simulink model "pacemaker"  (R2022b)
settings: Solver=FixedStepAuto  StartTime=0.0  StopTime=10.0  FixedStep=1e-3  RelTol=1e-3  EnableMultiTasking=on
undefined symbols (not defined in the file): a, A0, A1, b, c, D0, D1, D10, D11, D12, D13, D2, D3, D4, D5, D6, D7, D8, D9, PTA0, PTA1, PTA2, PTB2, PTB23, PTB3, PTB9, PTC16, PTC17, PTC2, PTC3, PTC4, PTD0, PTD1, PTD2, PTD3
libraries: frdmk64flib x21, simulink x2, etargetslib x2, dspstat3 x1, hdlsllib x1
settings Model: ExtModeTrigDuration=5  Creator=arnur  LastModifiedBy=arnur
settings SolverCC: AlgebraicLoopSolver=TrustRegion
settings OptimizationCC: EnhancedBackFolding=on  PassReuseOutputArgsAs=Individual arguments  ZeroExternalMemoryAtStartup=off  ZeroInternalMemoryAtStartup=off  MaxStackSize=64  OptimizeBlockOrder=speed  DifferentSizesBufferReuse=on  OptimizationCustomize=off  EfficientTunableParamExpr=on
settings DebuggingCC: ParameterTunabilityLossMsg=error  UnconnectedInputMsg=warning  UnconnectedOutputMsg=warning  UnconnectedLineMsg=warning
settings HardwareCC: ProdBitPerPointer=32  ProdBitPerSizeT=32  ProdBitPerPtrDiffT=32  ProdLargestAtomicInteger=Long  ProdLargestAtomicFloat=Double  ProdWordSize=32  ProdHWDeviceType=ARM Compatible->ARM Cortex
settings ModelReferenceCC: EnableRefExpFcnMdlSchedulingChecks=on
settings SFSimCC: MATLABDynamicMemAlloc=off
settings RTWCC: Description=Embedded Coder  SystemTargetFile=ert.tlc  HardwareBoard=NXP FRDM-K64F  TLCOptions="-aInlineSetEventsForThisBaseRateFcn=TLC_FALSE -aSuppressMultiTaskScheduler=TLC_FALSE  -aRateBasedStepFcn=0"  TemplateMakefile=ert_default_tmf  Toolchain=GNU Tools for ARM Embedded Processors
settings CodeAppCC: ForceParamTrailComments=on  IgnoreCustomStorageClasses=off  OperatorAnnotations=on  SimulinkDataObjDesc=on  SFDataObjDesc=on  InsertBlockDesc=on

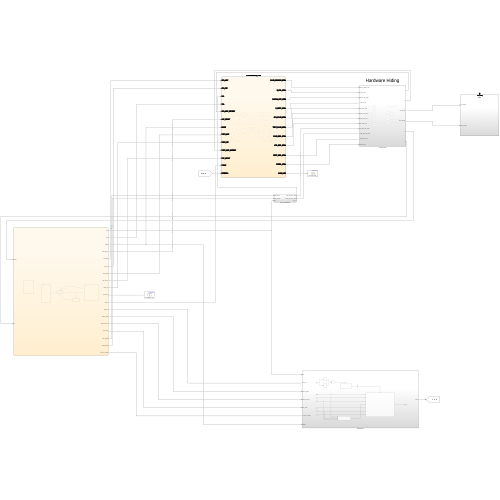
[thumbnail: Simulink's stored preview of the top-level diagram]
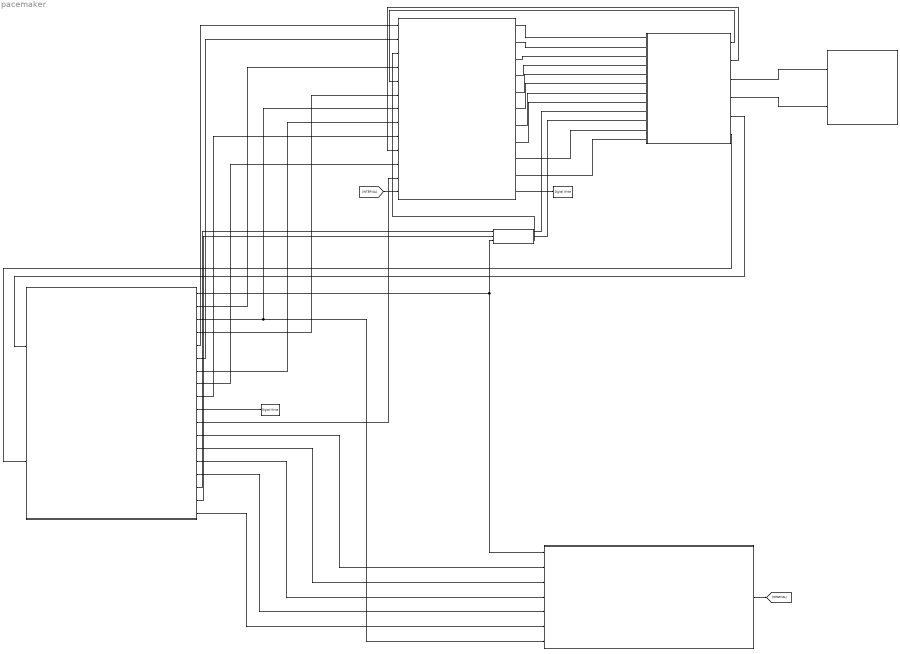
== system pacemaker ==
  note: Hardware Hiding
  Chart : Stateflow chart  TreatAsAtomicUnit=on
      settings: PortSchema="{\"entries\":[{\"content\":{\"sides\":[{\"content\":{\"connectorIds\":[\"In2\",\"In1\"]},\"type\":\"ConnectorPlacement.EquallySpacedRectSide\",\"uuid\":\"bc218187-1f13-41e7-927e-dd226419d8de\"},{\"content\":{\"connectorIds\":[\"Out1\",\"Out2\",\"Out3\",\"Out4\",\"Out5\",\"Out6\",\"Out7\",\"Out8\",\"Out9\",\"Out10\",\"Out11\",\"Out12\",\"Out13\",\"Out14\",\"Out15\",\"Out16\",\"Out17\",\"Out18\"],\"side\":\"RIGHT\"},\"type\":\"ConnectorPlacement.EquallySpacedRectSide\",\"uuid\":\"24412552-eff0-4bdb-8788-4cded0bceaa8\"},{\"content\":{\"connectorIds\":[],\"side\":\"TOP\"},\"type\":\"ConnectorPlacement.EquallySpacedRectSide\",\"uuid\":\"ae10373c-f6da-40d4-8510-ccb7acfbe125\"}]},\"type\":\"ConnectorPlacement.EquallySpacedConnector\",\"uuid\":\"32cdb14c-4a7f-42e8-a7b0-e0b40f5ef528\"}],\"packageUris\":[\"http://schema.mathworks.com/mf0/Connector/R2020b\"],\"version\":\"1.0\"}"
  Digital Write : frdmk64flib/Digital Write  Whichpin=GREEN_LED
  Digital Write1 : frdmk64flib/Digital Write  Whichpin=BLUE_LED
  Hardware Hiding : Subsystem
  INPUT_CONVERSION : Subsystem
  PACEMAKER_FSM : Stateflow chart  TreatAsAtomicUnit=on
  Rate Adaptivity : Subsystem
  Subsystem : Subsystem
  wires:
  Hardware Hiding/1(Output4) -> PACEMAKER_FSM/5(ATR_CMP_DETECT)
  Hardware Hiding/2(Output10) -> PACEMAKER_FSM/10(VENT_CMP_DETECT)
  Chart/5(ATR_AMP) -> PACEMAKER_FSM/1(ATR_AMP)
  Chart/9(VENT_PW) -> PACEMAKER_FSM/9(VENT_PW)
  Chart/8(VRP_DELAY) -> PACEMAKER_FSM/11(VRP_DELAY)
  PACEMAKER_FSM/2(Z_ATR_CTRL) -> Hardware Hiding/2(Z_ATR_CTRL)
  Chart/6(ATR_PW) -> PACEMAKER_FSM/2(ATR_PW)
  PACEMAKER_FSM/8(ATR_GND_CTRL) -> Hardware Hiding/8(ATR_GND_CTRL)
  Chart/7(VENT_AMP) -> PACEMAKER_FSM/8(VENT_AMP)
  Chart/1(LRL) -> INPUT_CONVERSION/3(LRL), Rate Adaptivity/1(LRL)
  Chart/2(URL) -> PACEMAKER_FSM/4(URL)
  PACEMAKER_FSM/5(ATR_PACE_CTRL) -> Hardware Hiding/5(ATR_PACE_CTRL)
  Chart/4(ARP_DELAY) -> PACEMAKER_FSM/6(ARP_DELAY)
  PACEMAKER_FSM/3(PACING_REF_PWM) -> Hardware Hiding/3(PACING_REF_PWM)
  PACEMAKER_FSM/6(VENT_PACE_CTRL) -> Hardware Hiding/6(VENT_PACE_CTRL)
  PACEMAKER_FSM/1(PACE_CHARGE_CTRL) -> Hardware Hiding/1(PACE_CHARGE_CTRL)
  Chart/3(MODE) -> PACEMAKER_FSM/7(MODE), Rate Adaptivity/7(MODE)
  PACEMAKER_FSM/9(VENT_GND_CTRL) -> Hardware Hiding/11(VENT_GND_CTRL)
  PACEMAKER_FSM/4(Z_VENT_CTRL) -> Hardware Hiding/4(Z_VENT_CTRL)
  PACEMAKER_FSM/7(PACE_GND_CTRL) -> Hardware Hiding/7(PACE_GND_CTRL)
  PACEMAKER_FSM/10(FRTND_CTRL) -> Hardware Hiding/12(FRTND_CTRL)
  Chart/10(green_LED) -> Digital Write/1
  Chart/11(PVARP) -> PACEMAKER_FSM/12(PVARP)
  Chart/12(MAX_SR) -> Rate Adaptivity/2(MAX_SR)
  Chart/13(REACT_TIME) -> Rate Adaptivity/3(REACT_TIME)
  Chart/14(RESP_FACTOR) -> Rate Adaptivity/4(RESP_FACTOR)
  Chart/15(REC_TIME) -> Rate Adaptivity/5(REC_TIME)
  Chart/16(ATR_SENSE) -> INPUT_CONVERSION/1(ATR_SENSE)
  Chart/17(VENT_SENSE) -> INPUT_CONVERSION/2(VENT_SENSE)
  Chart/18(ACTIVITY_THRES) -> Rate Adaptivity/6(ACTIVITY_THRES)
  Hardware Hiding/3(ATR_SIGNAL) -> Subsystem/1(ATR_SIGNAL)
  Hardware Hiding/4(VENT_SIGNAL) -> Subsystem/2(VENT_SIGNAL)
  INPUT_CONVERSION/1(ATR_CMP_REF_PWM) -> Hardware Hiding/9(ATR_CMP_REF_PWM)
  INPUT_CONVERSION/2(VENT_CMP_REF_PWM) -> Hardware Hiding/10(VENT_CMP_REF_PWM)
  Rate Adaptivity/1(interval) -> [INTERVAL]
  [INTERVAL] -> PACEMAKER_FSM/13(INTERVAL)
  PACEMAKER_FSM/11(BLUE_LED) -> Digital Write1/1
  INPUT_CONVERSION/3(LRL_P) -> PACEMAKER_FSM/3(LRL)
  Hardware Hiding/5(Output1) -> Chart/2(Status)
  Hardware Hiding/6(Output2) -> Chart/1(Rx)

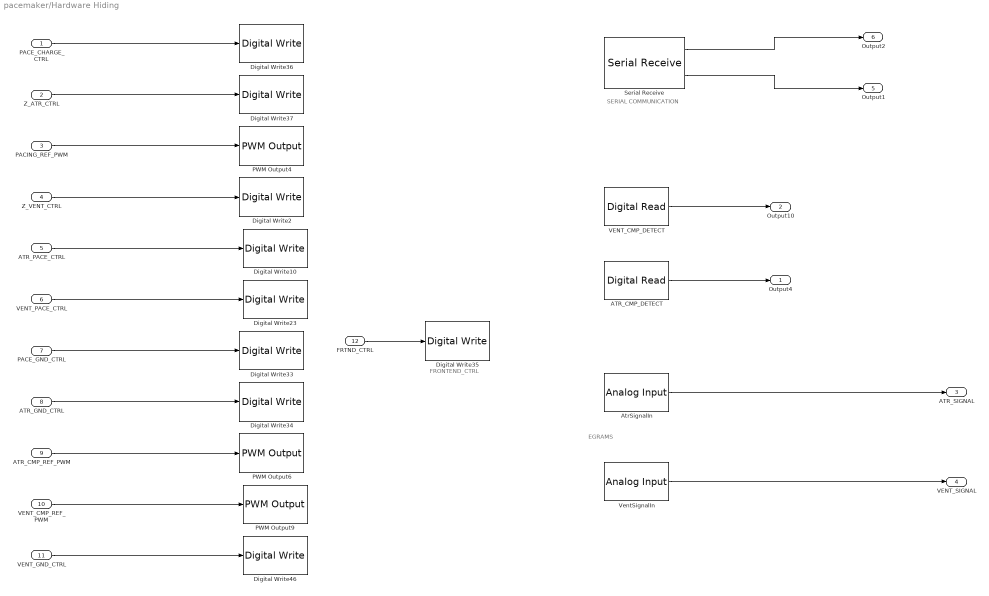
== system pacemaker/Hardware Hiding ==
  note: EGRAMS
  note: SERIAL COMMUNICATION
  note: FRONTEND_CTRL
  PACE_CHARGE_CTRL : Inport
  Z_ATR_CTRL : Inport  Port=2
  PACING_REF_PWM : Inport  Port=3
  Z_VENT_CTRL : Inport  Port=4
  ATR_PACE_CTRL : Inport  Port=5
  VENT_PACE_CTRL : Inport  Port=6
  PACE_GND_CTRL : Inport  Port=7
  ATR_GND_CTRL : Inport  Port=8
  ATR_CMP_REF_PWM : Inport  Port=9
  VENT_CMP_REF_PWM : Inport  Port=10
  VENT_GND_CTRL : Inport  Port=11
  FRTND_CTRL : Inport  Port=12  OutDataTypeStr=boolean  LockScale=on
  ATR_CMP_DETECT : frdmk64flib/Digital Read  Whichpin=PTC16 (D0)  SampleTime=-1
  AtrSignalIn : frdmk64flib/Analog Input  Whichpin=PTB2 (A0)  SampleTime=-1
  Digital Write10 : frdmk64flib/Digital Write  Whichpin=PTA0 (D8)
  Digital Write2 : frdmk64flib/Digital Write  Whichpin=PTC3 (D7)
  Digital Write23 : frdmk64flib/Digital Write  Whichpin=PTC4 (D9)
  Digital Write33 : frdmk64flib/Digital Write  Whichpin=PTD0 (D10)
  Digital Write34 : frdmk64flib/Digital Write  Whichpin=PTD2 (D11)
  Digital Write35 : frdmk64flib/Digital Write  Whichpin=PTD1 (D13)
  Digital Write36 : frdmk64flib/Digital Write  Whichpin=PTB9 (D2)
  Digital Write37 : frdmk64flib/Digital Write  Whichpin=PTB23 (D4)
  Digital Write46 : frdmk64flib/Digital Write  Whichpin=PTD3 (D12)
  PWM Output4 : frdmk64flib/PWM Output  Whichpin=PTA2 (D5)  InitialFrequency=2000  InitialDutyCycle=0
  PWM Output6 : frdmk64flib/PWM Output  Whichpin=PTC2 (D6)  InitialFrequency=2000  InitialDutyCycle=0
  PWM Output9 : frdmk64flib/PWM Output  Whichpin=PTA1 (D3)  InitialFrequency=2000  InitialDutyCycle=0
  Serial Receive : frdmk64flib/Serial Receive  SCIModule=0  Baudrate=uint32(9600)  Parity=None  StopBits=1  HardwareFlowControl=None  ByteOrder=LittleEndian  DataType=uint8  DataLength=49  BlockingMode=off  OutputStatus=on  SampleTime=-1
  VENT_CMP_DETECT : frdmk64flib/Digital Read  Whichpin=PTC17 (D1)  SampleTime=-1
  VentSignalIn : frdmk64flib/Analog Input  Whichpin=PTB3 (A1)  SampleTime=-1
  Output4 : Outport
  Output10 : Outport  Port=2
  ATR_SIGNAL : Outport  Port=3
  VENT_SIGNAL : Outport  Port=4
  Output1 : Outport  Port=5
  Output2 : Outport  Port=6
  wires:
  VENT_GND_CTRL/1 -> Digital Write46/1
  Z_VENT_CTRL/1 -> Digital Write2/1
  VENT_PACE_CTRL/1 -> Digital Write23/1
  ATR_CMP_REF_PWM/1 -> PWM Output6/1
  VENT_CMP_REF_PWM/1 -> PWM Output9/1
  PACE_CHARGE_CTRL/1 -> Digital Write36/1
  Z_ATR_CTRL/1 -> Digital Write37/1
  ATR_PACE_CTRL/1 -> Digital Write10/1
  PACE_GND_CTRL/1 -> Digital Write33/1
  ATR_GND_CTRL/1 -> Digital Write34/1
  PACING_REF_PWM/1 -> PWM Output4/1
  ATR_CMP_DETECT/1 -> Output4/1
  VENT_CMP_DETECT/1 -> Output10/1
  FRTND_CTRL/1 -> Digital Write35/1
  VentSignalIn/1 -> VENT_SIGNAL/1
  AtrSignalIn/1 -> ATR_SIGNAL/1
  Serial Receive/1 -> Output2/1
  Serial Receive/2 -> Output1/1

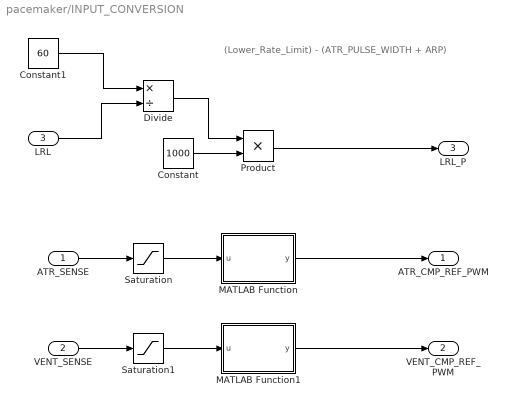
== system pacemaker/INPUT_CONVERSION ==
  note: (Lower_Rate_Limit) - (ATR_PULSE_WIDTH + ARP)
  ATR_SENSE : Inport
  VENT_SENSE : Inport  Port=2
  LRL : Inport  Port=3  OutDataTypeStr=uint16
  Constant : Constant  Value=1000  OutDataTypeStr=double
  Constant1 : Constant  Value=60  OutDataTypeStr=double
  Divide : Product  Inputs=*/  OutDataTypeStr=double
  MATLAB Function : MATLAB Function  TreatAsAtomicUnit=on
  MATLAB Function1 : MATLAB Function  TreatAsAtomicUnit=on
  Product : Product  OutDataTypeStr=double
  Saturation : Saturate  UpperLimit=4  LowerLimit=0.65  OutDataTypeStr=double
  Saturation1 : Saturate  UpperLimit=4  LowerLimit=0.65  OutDataTypeStr=double
  ATR_CMP_REF_PWM : Outport
  VENT_CMP_REF_PWM : Outport  Port=2
  LRL_P : Outport  Port=3  OutDataTypeStr=double
  wires:
  ATR_SENSE/1 -> Saturation/1
  Saturation/1 -> MATLAB Function/1(u)
  MATLAB Function/1(y) -> ATR_CMP_REF_PWM/1
  MATLAB Function1/1(y) -> VENT_CMP_REF_PWM/1
  VENT_SENSE/1 -> Saturation1/1
  Saturation1/1 -> MATLAB Function1/1(u)
  Product/1 -> LRL_P/1
  Constant/1 -> Product/2
  LRL/1 -> Divide/2
  Divide/1 -> Product/1
  Constant1/1 -> Divide/1

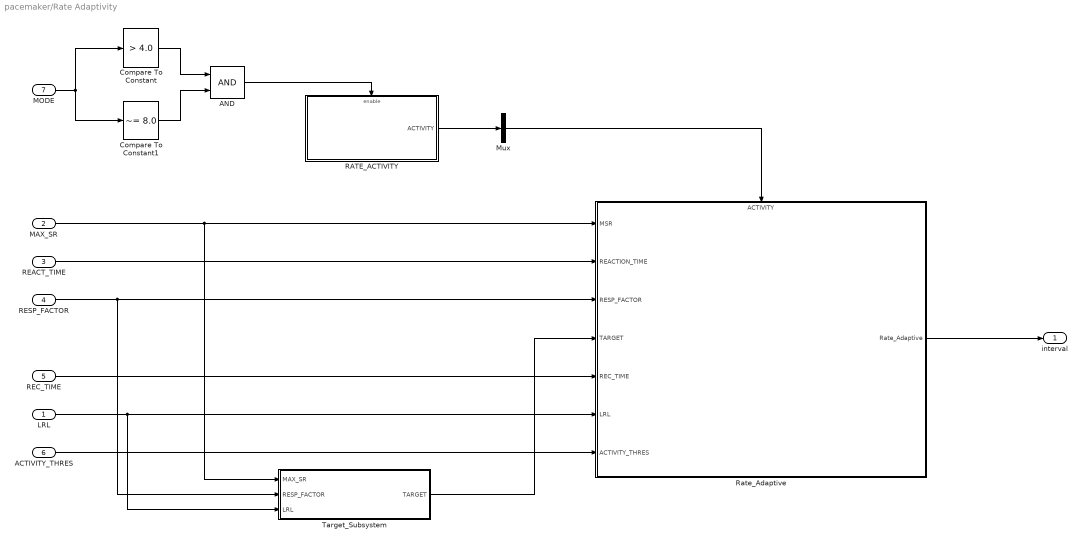
== system pacemaker/Rate Adaptivity ==
  LRL : Inport
  MAX_SR : Inport  Port=2
  REACT_TIME : Inport  Port=3
  RESP_FACTOR : Inport  Port=4
  REC_TIME : Inport  Port=5
  ACTIVITY_THRES : Inport  Port=6  OutDataTypeStr=double
  MODE : Inport  Port=7
  AND : Logic  IconShape=distinctive  AllPortsSameDT=off  OutDataTypeStr=boolean
  Compare To Constant : simulink/Logic and Bit Operations/Compare To Constant  relop=>  const=4.0  OutDataTypeStr=boolean
  Compare To Constant1 : simulink/Logic and Bit Operations/Compare To Constant  relop=~=  const=8.0  OutDataTypeStr=boolean
  Mux : Mux  Inputs=1
  RATE_ACTIVITY : Subsystem
  Rate_Adaptive : Subsystem
      settings: PortSchema="{\"entries\":[{\"content\":{\"sides\":[{\"content\":{\"connectorIds\":[\"In1\",\"In2\",\"In3\",\"In4\",\"In5\",\"In6\",\"In7\"]},\"type\":\"ConnectorPlacement.EquallySpacedRectSide\",\"uuid\":\"ecef5992-6168-4615-8079-152f4001d897\"},{\"content\":{\"connectorIds\":[\"Out1\"],\"side\":\"RIGHT\"},\"type\":\"ConnectorPlacement.EquallySpacedRectSide\",\"uuid\":\"4b0443a4-3c4f-432b-8acf-b8853e3911f3\"},{\"content\":{\"connectorIds\":[\"In8\"],\"side\":\"TOP\"},\"type\":\"ConnectorPlacement.EquallySpacedRectSide\",\"uuid\":\"9eb25122-da38-4088-8f00-2d2dff5efbee\"},{\"content\":{\"connectorIds\":[],\"side\":\"BOTTOM\"},\"type\":\"ConnectorPlacement.EquallySpacedRectSide\",\"uuid\":\"f562ad64-64af-4bdb-b61f-82ac1a60a400\"}]},\"type\":\"ConnectorPlacement.EquallySpacedConnector\",\"uuid\":\"02b21474-b9be-4120-8392-47ed1544c592\"}],\"packageUris\":[\"http://schema.mathworks.com/mf0/Connector/R2020b\"],\"version\":\"1.0\"}"
  Target_Subsystem : Subsystem
  interval : Outport
  wires:
  REC_TIME/1 -> Rate_Adaptive/5(REC_TIME)
  Target_Subsystem/1(TARGET) -> Rate_Adaptive/4(TARGET)
  REACT_TIME/1 -> Rate_Adaptive/2(REACTION_TIME)
  Rate_Adaptive/1(Rate_Adaptive) -> interval/1
  RESP_FACTOR/1 -> Rate_Adaptive/3(RESP_FACTOR), Target_Subsystem/2(RESP_FACTOR)
  LRL/1 -> Target_Subsystem/3(LRL), Rate_Adaptive/6(LRL)
  MAX_SR/1 -> Target_Subsystem/1(MAX_SR), Rate_Adaptive/1(MSR)
  ACTIVITY_THRES/1 -> Rate_Adaptive/7(ACTIVITY_THRES)
  AND/1 -> RATE_ACTIVITY/Enable
  Mux/1 -> Rate_Adaptive/8(ACTIVITY)
  Compare To Constant/1 -> AND/1
  Compare To Constant1/1 -> AND/2
  RATE_ACTIVITY/1(ACTIVITY) -> Mux/1
  MODE/1 -> Compare To Constant1/1, Compare To Constant/1

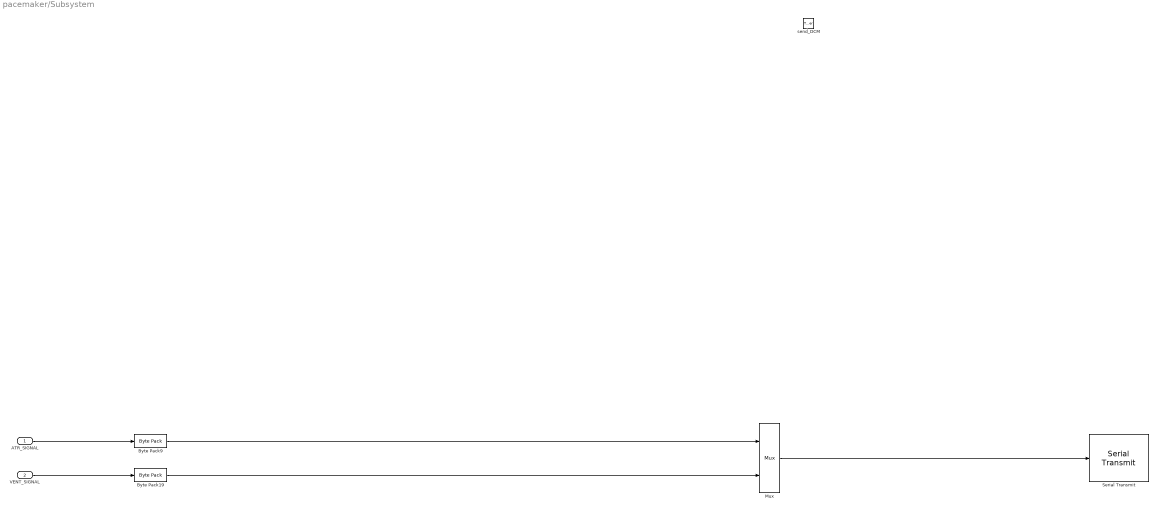
== system pacemaker/Subsystem ==
  ATR_SIGNAL : Inport
  VENT_SIGNAL : Inport  Port=2
  send_DCM : TriggerPort  TriggerType=function-call  IsSimulinkFunction=on  FunctionName=send_DCM  VariantControl=Variant
  Byte Pack19 : etargetslib/Byte Pack  datatypes={'double'}  byteAlign=1
  Byte Pack9 : etargetslib/Byte Pack  datatypes={'double'}  byteAlign=1
  Mux : Mux  Inputs=2
  Serial Transmit : frdmk64flib/Serial Transmit  SCIModule=0  Baudrate=uint32(9600)  Parity=None  StopBits=1  HardwareFlowControl=None  ByteOrder=LittleEndian  BlockingMode=on  OutputStatus=off
  wires:
  Mux/1 -> Serial Transmit/1
  ATR_SIGNAL/1 -> Byte Pack9/1
  VENT_SIGNAL/1 -> Byte Pack19/1
  Byte Pack9/1 -> Mux/1
  Byte Pack19/1 -> Mux/2

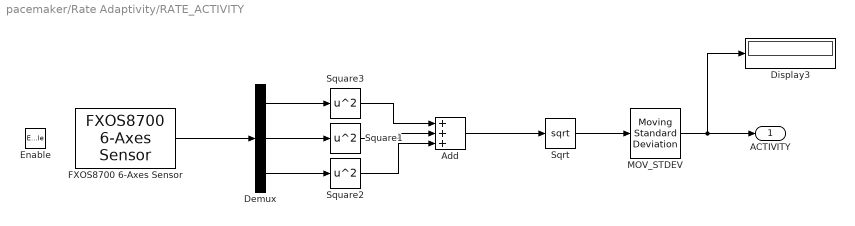
== system pacemaker/Rate Adaptivity/RATE_ACTIVITY ==
  Enable : EnablePort
  Add : Sum  Inputs=+++
  Demux : Demux  Outputs=3
  Display3 : Display
  FXOS8700 6-Axes Sensor : frdmk64flib/FXOS8700 6-Axes Sensor  Activesensor=Accelerometer only  ODR=800Hz  HybridODR=400Hz  Accelfullrange=-4g to +4g  SampleTime=-1
  MOV_STDEV : dspstat3/Moving Standard Deviation  Method=Sliding window  ForgettingFactorPort=off  SpecifyWindowLength=on  WindowLength=156  OverlapLength=155  AllowArbitraryInputLength=off  ForgettingFactor=0.9  SimulateUsing=Code generation
  Sqrt : Sqrt
  Square1 : Math  Operator=square  OutDataTypeStr=double
  Square2 : Math  Operator=square  OutDataTypeStr=double
  Square3 : Math  Operator=square  OutDataTypeStr=double
  ACTIVITY : Outport
  wires:
  FXOS8700 6-Axes Sensor/1 -> Demux/1
  Demux/3 -> Square2/1
  Square1/1 -> Add/2
  Add/1 -> Sqrt/1
  Demux/2 -> Square1/1
  Square3/1 -> Add/1
  Square2/1 -> Add/3
  Demux/1 -> Square3/1
  Sqrt/1 -> MOV_STDEV/1
  MOV_STDEV/1 -> Display3/1, ACTIVITY/1

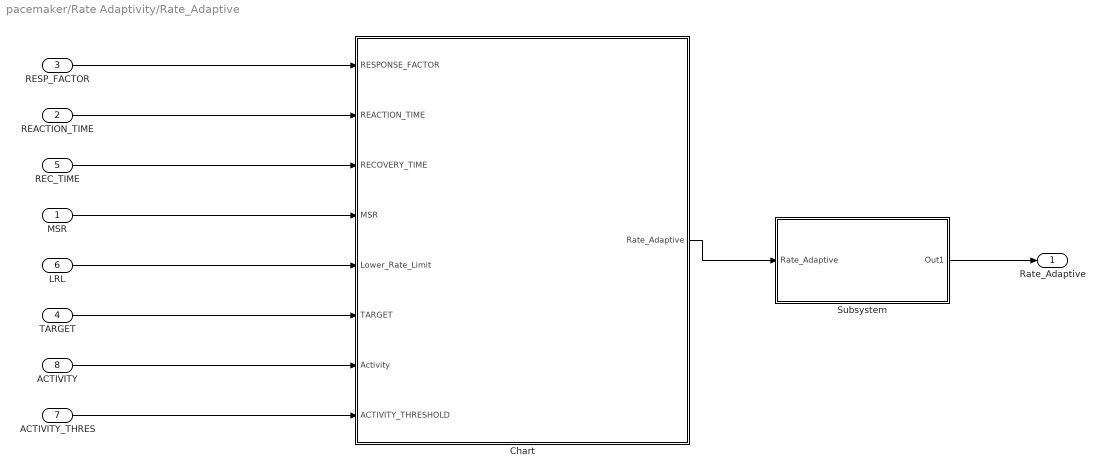
== system pacemaker/Rate Adaptivity/Rate_Adaptive ==
  MSR : Inport
  REACTION_TIME : Inport  Port=2
  RESP_FACTOR : Inport  Port=3
  TARGET : Inport  Port=4
  REC_TIME : Inport  Port=5
  LRL : Inport  Port=6
  ACTIVITY_THRES : Inport  Port=7
  ACTIVITY : Inport  Port=8
  Chart : Stateflow chart  TreatAsAtomicUnit=on
  Subsystem : Subsystem
  Rate_Adaptive : Outport
  wires:
  RESP_FACTOR/1 -> Chart/1(RESPONSE_FACTOR)
  REACTION_TIME/1 -> Chart/2(REACTION_TIME)
  REC_TIME/1 -> Chart/3(RECOVERY_TIME)
  ACTIVITY_THRES/1 -> Chart/8(ACTIVITY_THRESHOLD)
  MSR/1 -> Chart/4(MSR)
  LRL/1 -> Chart/5(Lower_Rate_Limit)
  TARGET/1 -> Chart/6(TARGET)
  ACTIVITY/1 -> Chart/7(Activity)
  Chart/1(Rate_Adaptive) -> Subsystem/1(Rate_Adaptive)
  Subsystem/1(Out1) -> Rate_Adaptive/1

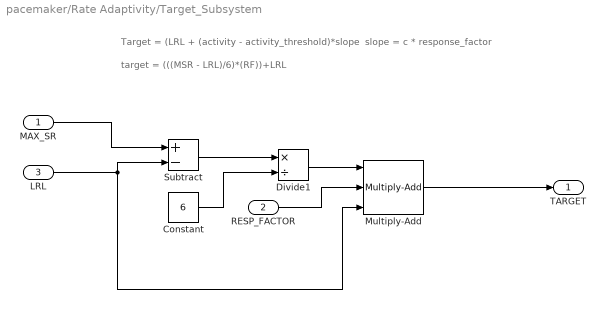
== system pacemaker/Rate Adaptivity/Target_Subsystem ==
  note: target = (((MSR - LRL)/6)*(RF))+LRL
  note: slope = c * response_factor
  note: Target = (LRL + (activity - activity_threshold)*slope
  MAX_SR : Inport
  RESP_FACTOR : Inport  Port=2
  LRL : Inport  Port=3
  Constant : Constant  Value=6
  Divide1 : Product  Inputs=*/
  Multiply-Add : hdlsllib/HDL Operations/Multiply-Add  Function=c+(a.*b)  datatype=uint16  RndMeth=Round  DoSatur=off  FMA=off
  Subtract : Sum  Inputs=+-
  TARGET : Outport  OutDataTypeStr=uint16
  wires:
  RESP_FACTOR/1 -> Multiply-Add/2
  Constant/1 -> Divide1/2
  MAX_SR/1 -> Subtract/1
  LRL/1 -> Subtract/2, Multiply-Add/3
  Divide1/1 -> Multiply-Add/1
  Multiply-Add/1 -> TARGET/1
  Subtract/1 -> Divide1/1

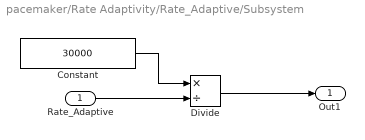
== system pacemaker/Rate Adaptivity/Rate_Adaptive/Subsystem ==
  Rate_Adaptive : Inport
  Constant : Constant  Value=30000  OutDataTypeStr=uint16
  Divide : Product  Inputs=*/
  Out1 : Outport  OutDataTypeStr=uint16
  wires:
  Constant/1 -> Divide/1
  Rate_Adaptive/1 -> Divide/2
  Divide/1 -> Out1/1

== matlab function pacemaker/INPUT_CONVERSION/MATLAB Function1 ==
  data: u input; y output
function y = fcn(u)

y = u./5.*100;

== matlab function pacemaker/INPUT_CONVERSION/MATLAB Function ==
  data: u input; y output
function y = fcn(u)

y = u./5.*100;

== stateflow chart pacemaker/Chart ==
  note: MODE
      | AOO: 1
      | AAI: 2
      | VVO: 3
      | VVI: 4
      | %RATE ADAPTIVE
      | AOOR: 5
      | AAIR: 6
      | VOOR: 7
      | VVIR: 8
  state INITIAL
    %initializing parameters
    entry:
    MODE = 5;
    LRL = 60;
    URL = 120;
    ARP_DELAY  =200;
    ATR_AMP = 3.5;
    VENT_AMP= 3.5;
    VRP_DELAY= 200;
    ATR_PW= 10;
    VENT_PW = 10;
    %
    PVARP = 200% uint_16
    MAX_SR = 120 % uint_16
    REACT_TIME = 30 %uint_8
    RESP_FACTOR = 16 %uint_8
    REC_TIME = 2 %uint_8
    ATR_SENSE = 3 %single
    VENT_SENSE = 3%single
    ACTIVITY_THRES = 0.2 % uint_8
    %
    green_LED = false;
  state SET_PARAM
    entry:
    MODE = typecast(Rx(3),'uint8');
    LRL = typecast(Rx(4:5),'uint16');
    URL =typecast(Rx(6:7),'uint16');
    ARP_DELAY  = typecast(Rx(8:9),'uint16');
    ATR_AMP = typecast(Rx(10:13),'single');
    VENT_AMP= typecast(Rx(14:17),'single');
    VRP_DELAY= typecast(Rx(18:19),'uint16');
    ATR_PW= typecast(Rx(20:21),'uint16');
    VENT_PW = typecast(Rx(22:23),'uint16');
    ATR_SENSE = typecast(Rx(24:27), 'single');
    VENT_SENSE = typecast(Rx(28:31), 'single');
    PVARP = typecast(Rx(32:33), 'uint16');
    MAX_SR = typecast(Rx(34:35), 'uint16');
    REACT_TIME = typecast(Rx(36:37),'uint16');
    RESP_FACTOR =  typecast(Rx(38:39),'uint16');
    REC_TIME =  typecast(Rx(40:41),'uint16');
    ACTIVITY_THRES =  typecast(Rx(42:49),'double');
    green_LED = false;
  state STANDBY
    % Wait for the inputs
  state ECHO_PARAM
    entry:
    send_DCM();
    green_LED = false;
  (default) -> INITIAL
  SET_PARAM -> STANDBY
  (junction 33) -> STANDBY [order 2]
  INITIAL -> STANDBY
  STANDBY -> (junction 33) : [Status==0]
  (junction 33) -> (junction 36) [order 1] : [Rx(1)==hex2dec('16')]
  (junction 36) -> SET_PARAM [order 2] : [Rx(2) == hex2dec('12')]
  (junction 36) -> ECHO_PARAM [order 1] : [Rx(2) == hex2dec('22')]
  ECHO_PARAM -> STANDBY
  data: Rx input uint8; Status input uint8 size=1; LRL output uint16; URL output uint16; MODE output uint8; ARP_DELAY output uint16; ATR_AMP output single; ATR_PW output uint16; VENT_AMP output single; VRP_DELAY output uint16; VENT_PW output uint16; green_LED output boolean; PVARP output uint16; MAX_SR output uint16; REACT_TIME output uint16; RESP_FACTOR output uint16; REC_TIME output uint16; ATR_SENSE output single; VENT_SENSE output single; ACTIVITY_THRES output double

== stateflow chart pacemaker/Rate Adaptivity/Rate_Adaptive/Chart ==
  state State1
    entry:
    Rate_Adaptive = Lower_Rate_Limit;
    %when activity is less than activity threshold the rate adaptive is equal to LRL
  state State3
    entry:
    Rate_Adaptive = TARGET;
    %If activity is continued then the rate adaptive will eventually reach the target rate
  state State2
    entry:
    Rate_Adaptive = Rate_Adaptive + Step_Up;
    %Rate adaptive is calculated using step size when activity is high
  state State5
    entry:
    Rate_Adaptive = Rate_Adaptive - Step_Down;
    %continue to decrease rate adaptive until LRL is reached
  state State4
    entry:
    Rate_Adaptive = Rate_Adaptive - Step_Up;
    %once the activty starts decreasing we need to decrease rate adaptive
  (default) -> State1 : {Step_Up = ceil((TARGET - Lower_Rate_Limit)/REACTION_TIME);
      | Step_Down = ceil((TARGET - Lower_Rate_Limit)/RECOVERY_TIME)}
  State1 -> State1 [order 1] : [Activity < ACTIVITY_THRESHOLD]
  State2 -> State2 [order 2] : after(1000,msec)[Rate_Adaptive <= TARGET]
  State3 -> State3 [order 2] : [Activity > ACTIVITY_THRESHOLD]
  State1 -> State2 [order 2] : [Activity >= ACTIVITY_THRESHOLD]
  State2 -> State3 [order 3] : [Rate_Adaptive >= TARGET]
  State3 -> State5 [order 1] : [Activity < ACTIVITY_THRESHOLD]
  State5 -> State1 [order 1] : [Rate_Adaptive <= Lower_Rate_Limit]
  State5 -> State2 [order 3] : [Activity >= ACTIVITY_THRESHOLD]
  State2 -> State4 [order 1] : [Activity < ACTIVITY_THRESHOLD]
  State4 -> State2 [order 1] : [Activity >= ACTIVITY_THRESHOLD]
  State4 -> State5 [order 2] : [after(1000,msec)]
  State5 -> State5 [order 2] : after(1000,msec)[Rate_Adaptive >= Lower_Rate_Limit]
  data: RESPONSE_FACTOR input; REACTION_TIME input; RECOVERY_TIME input; MSR input; Lower_Rate_Limit input; TARGET input; Activity input; ACTIVITY_THRESHOLD input; Rate_Adaptive output; Step_Up local uint16; Step_Down local uint16

== stateflow chart pacemaker/PACEMAKER_FSM ==
  note: VOOR
  note: AOOR
  state Charging_C22_and_Discharging_Blocking_Cap4
    entry:
    FRTND_CTRL= true;
    ATR_PACE_CTRL = false;
    VENT_PACE_CTRL= false;
    PACING_REF_PWM = (ATR_AMP*100)/5;
    PACE_CHARGE_CTRL = true;
    PACE_GND_CTRL = true;
    Z_ATR_CTRL = false;
    Z_VENT_CTRL = false;
    ATR_GND_CTRL = true;
    FRTND_CTRL= true;
    BLUE_LED = false;
  state Charging_C22_and_Discharging_Blocking_Cap5
    entry:
    ATR_PACE_CTRL = false;
    VENT_PACE_CTRL= false;
    PACING_REF_PWM = (VENT_AMP*100)/5;
    PACE_CHARGE_CTRL = true;
    PACE_GND_CTRL = true;
    Z_ATR_CTRL = false;
    Z_VENT_CTRL = false;
    %ATR_GND_CTRL = true;
    VENT_GND_CTRL = true;
  state Discharging_C22_into_AV__charge_C26
    entry:
    PACE_CHARGE_CTRL = false;
    PACE_GND_CTRL = true;
    ATR_PACE_CTRL = false;
    %ATR_GND_CTRL = false;
    Z_ATR_CTRL = false;
    Z_VENT_CTRL = false;
    VENT_GND_CTRL = false;
    VENT_PACE_CTRL = true;
  state Discharging_C22_into_AV__charge_C25
    entry:
    FRTND_CTRL= false;
    PACE_CHARGE_CTRL = false;
    PACE_GND_CTRL = true;
    ATR_PACE_CTRL = true;
    ATR_GND_CTRL = false;
    Z_ATR_CTRL = false;
    Z_VENT_CTRL = false;
    VENT_PACE_CTRL = false;
    FRTND_CTRL= false;
    BLUE_LED = true;
  note: VOO
  note: AOO
  state Charging_C22_and_Discharging_Blocking_Cap3
    entry:
    ATR_PACE_CTRL = false;
    VENT_PACE_CTRL= false;
    PACING_REF_PWM = (VENT_AMP*100)/5;
    PACE_CHARGE_CTRL = true;
    PACE_GND_CTRL = true;
    Z_ATR_CTRL = false;
    Z_VENT_CTRL = false;
    %ATR_GND_CTRL = true;
    VENT_GND_CTRL = true;
  state Discharging_C22_into_AV__charge_C24
    entry:
    PACE_CHARGE_CTRL = false;
    PACE_GND_CTRL = true;
    ATR_PACE_CTRL = false;
    %ATR_GND_CTRL = false;
    Z_ATR_CTRL = false;
    Z_VENT_CTRL = false;
    VENT_GND_CTRL = false;
    VENT_PACE_CTRL = true;
  state Charging_C22_and_Discharging_Blocking_Cap
    entry:
    ATR_PACE_CTRL = false;
    VENT_PACE_CTRL= false;
    PACING_REF_PWM = (ATR_AMP*100)/5;
    PACE_CHARGE_CTRL = true;
    PACE_GND_CTRL = true;
    Z_ATR_CTRL = false;
    Z_VENT_CTRL = false;
    ATR_GND_CTRL = true;
    BLUE_LED = false;
  state Discharging_C22_into_AV__charge_C21
    entry:
    PACE_CHARGE_CTRL = false;
    PACE_GND_CTRL = true;
    ATR_PACE_CTRL = true;
    ATR_GND_CTRL = false;
    Z_ATR_CTRL = false;
    Z_VENT_CTRL = false;
    VENT_PACE_CTRL = false;
    BLUE_LED = true;
  state Initial
    entry:
    BLUE_LED = true;
    FRTND_CTRL= false;
  note: AAI
  note: VVI
  state Charging_C22_and_Discharging_Blocking_Cap2
    entry:
    ATR_PACE_CTRL = false;
    VENT_PACE_CTRL= false;
    PACING_REF_PWM = (VENT_AMP*100)/5;
    PACE_CHARGE_CTRL = true;
    PACE_GND_CTRL = true;
    Z_ATR_CTRL = false;
    Z_VENT_CTRL = false;
    %ATR_GND_CTRL = true;
    VENT_GND_CTRL = true;
    FRTND_CTRL= true;
  state Discharging_C22_into_AV__charge_C23
    entry:
    PACE_CHARGE_CTRL = false;
    PACE_GND_CTRL = true;
    ATR_PACE_CTRL = false;
    %ATR_GND_CTRL = false;
    Z_ATR_CTRL = false;
    Z_VENT_CTRL = false;
    VENT_GND_CTRL = false;
    VENT_PACE_CTRL = true;
  state Charging_C22_and_Discharging_Blocking_Cap1
    entry:
    ATR_PACE_CTRL = false;
    VENT_PACE_CTRL= false;
    PACING_REF_PWM = (ATR_AMP*100)/5;
    PACE_CHARGE_CTRL = true;
    PACE_GND_CTRL = true;
    Z_ATR_CTRL = false;
    Z_VENT_CTRL = false;
    ATR_GND_CTRL = true;
    FRTND_CTRL= true;
  state Discharging_C22_into_AV__charge_C22
    entry:
    PACE_CHARGE_CTRL = false;
    PACE_GND_CTRL = true;
    ATR_PACE_CTRL = true;
    ATR_GND_CTRL = false;
    Z_ATR_CTRL = false;
    Z_VENT_CTRL = false;
    VENT_PACE_CTRL = false;
  note: VVIR
  state Charging_C22_and_Discharging_Blocking_Cap6
    entry:
    ATR_PACE_CTRL = false;
    VENT_PACE_CTRL= false;
    PACING_REF_PWM = (ATR_AMP*100)/5;
    PACE_CHARGE_CTRL = true;
    PACE_GND_CTRL = true;
    Z_ATR_CTRL = false;
    Z_VENT_CTRL = false;
    ATR_GND_CTRL = true;
    FRTND_CTRL= true;
  state Charging_C22_and_Discharging_Blocking_Cap7
    entry:
    ATR_PACE_CTRL = false;
    VENT_PACE_CTRL= false;
    PACING_REF_PWM = (VENT_AMP*100)/5;
    PACE_CHARGE_CTRL = true;
    PACE_GND_CTRL = true;
    Z_ATR_CTRL = false;
    Z_VENT_CTRL = false;
    %ATR_GND_CTRL = true;
    VENT_GND_CTRL = true;
    FRTND_CTRL= true;
  state Discharging_C22_into_AV__charge_C28
    entry:
    PACE_CHARGE_CTRL = false;
    PACE_GND_CTRL = true;
    ATR_PACE_CTRL = false;
    %ATR_GND_CTRL = false;
    Z_ATR_CTRL = false;
    Z_VENT_CTRL = false;
    VENT_GND_CTRL = false;
    VENT_PACE_CTRL = true;
  state Discharging_C22_into_AV__charge_C27
    entry:
    PACE_CHARGE_CTRL = false;
    PACE_GND_CTRL = true;
    ATR_PACE_CTRL = true;
    ATR_GND_CTRL = false;
    Z_ATR_CTRL = false;
    Z_VENT_CTRL = false;
    VENT_PACE_CTRL = false;
  note: AAIR
  Charging_C22_and_Discharging_Blocking_Cap4 -> Discharging_C22_into_AV__charge_C25 : [after ((INTERVAL - ATR_PW ),msec)]
  Charging_C22_and_Discharging_Blocking_Cap5 -> Discharging_C22_into_AV__charge_C26 : [after ((INTERVAL - VENT_PW ),msec)]
  Discharging_C22_into_AV__charge_C26 -> Initial [order 2] : [MODE~=7]
  Discharging_C22_into_AV__charge_C26 -> Charging_C22_and_Discharging_Blocking_Cap5 [order 1] : [after(VENT_PW,msec)]
  Initial -> Charging_C22_and_Discharging_Blocking_Cap4 [order 5] : [MODE==5]
  Discharging_C22_into_AV__charge_C25 -> Charging_C22_and_Discharging_Blocking_Cap4 [order 2] : [after(ATR_PW,msec)]
  Initial -> Charging_C22_and_Discharging_Blocking_Cap5 [order 1] : [MODE==7]
  Discharging_C22_into_AV__charge_C25 -> Initial [order 1] : [MODE~=5]
  Discharging_C22_into_AV__charge_C21 -> Initial [order 2] : [MODE~=1]
  Initial -> Discharging_C22_into_AV__charge_C24 [order 8] : [MODE==3]
  Charging_C22_and_Discharging_Blocking_Cap3 -> Discharging_C22_into_AV__charge_C24 : [after ((LRL - VENT_PW ),msec)]
  Charging_C22_and_Discharging_Blocking_Cap -> Discharging_C22_into_AV__charge_C21 : [after ((LRL - ATR_PW ),msec)]
  Discharging_C22_into_AV__charge_C24 -> Charging_C22_and_Discharging_Blocking_Cap3 [order 1] : [after(VENT_PW,msec)]
  Initial -> Charging_C22_and_Discharging_Blocking_Cap [order 2] : [MODE==1]
  (default) -> Initial
  Discharging_C22_into_AV__charge_C21 -> Charging_C22_and_Discharging_Blocking_Cap [order 1] : [after(ATR_PW,msec)]
  Discharging_C22_into_AV__charge_C24 -> Initial [order 2] : [MODE~=3]
  Initial -> Charging_C22_and_Discharging_Blocking_Cap2 [order 7] : [MODE==4]
  Discharging_C22_into_AV__charge_C28 -> Initial [order 2] : [MODE~=8]
  Discharging_C22_into_AV__charge_C23 -> Initial [order 2] : [MODE~=4]
  Initial -> Charging_C22_and_Discharging_Blocking_Cap7 [order 3] : [MODE==8]
  Discharging_C22_into_AV__charge_C27 -> Initial [order 2] : [MODE~=6]
  Initial -> Charging_C22_and_Discharging_Blocking_Cap6 [order 4] : [MODE==6]
  Discharging_C22_into_AV__charge_C22 -> Initial [order 2] : [MODE~=2]
  Initial -> Charging_C22_and_Discharging_Blocking_Cap1 [order 6] : [MODE==2]
  Charging_C22_and_Discharging_Blocking_Cap1 -> Discharging_C22_into_AV__charge_C22 [order 1] : [after ((LRL - ATR_PW),msec) ]
  Discharging_C22_into_AV__charge_C23 -> Charging_C22_and_Discharging_Blocking_Cap2 [order 1] : [after(VENT_PW,msec)]
  Charging_C22_and_Discharging_Blocking_Cap1 -> Charging_C22_and_Discharging_Blocking_Cap1 [order 2] : [after(ARP_DELAY,msec) && ATR_CMP_DETECT == true]
  Discharging_C22_into_AV__charge_C22 -> Charging_C22_and_Discharging_Blocking_Cap1 [order 1] : [after(ATR_PW,msec)]
  Charging_C22_and_Discharging_Blocking_Cap2 -> Discharging_C22_into_AV__charge_C23 [order 2] : [after ((LRL - VENT_PW),msec) ]
  Charging_C22_and_Discharging_Blocking_Cap2 -> Charging_C22_and_Discharging_Blocking_Cap2 [order 1] : [after(VRP_DELAY,msec) && VENT_CMP_DETECT == true]
  Charging_C22_and_Discharging_Blocking_Cap6 -> Discharging_C22_into_AV__charge_C27 [order 1] : [after ((INTERVAL - ATR_PW),msec) ]
  Discharging_C22_into_AV__charge_C28 -> Charging_C22_and_Discharging_Blocking_Cap7 [order 1] : [after(VENT_PW,msec)]
  Charging_C22_and_Discharging_Blocking_Cap6 -> Charging_C22_and_Discharging_Blocking_Cap6 [order 2] : [after(ARP_DELAY,msec) && ATR_CMP_DETECT == true]
  Discharging_C22_into_AV__charge_C27 -> Charging_C22_and_Discharging_Blocking_Cap6 [order 1] : [after(ATR_PW,msec)]
  Charging_C22_and_Discharging_Blocking_Cap7 -> Discharging_C22_into_AV__charge_C28 [order 2] : [after ((LRL - VENT_PW),msec) ]
  Charging_C22_and_Discharging_Blocking_Cap7 -> Charging_C22_and_Discharging_Blocking_Cap7 [order 1] : [after(VRP_DELAY,msec) && VENT_CMP_DETECT == true]
  data: PACE_CHARGE_CTRL output; Z_ATR_CTRL output; PACING_REF_PWM output; Z_VENT_CTRL output; ATR_PACE_CTRL output; VENT_PACE_CTRL output; PACE_GND_CTRL output; ATR_GND_CTRL output; ATR_AMP input; ATR_PW input; LRL input; URL input; ATR_CMP_DETECT input; ARP_DELAY input; MODE input uint8; VENT_AMP input; VENT_PW input; VENT_CMP_DETECT input; VRP_DELAY input; VENT_GND_CTRL output; FRTND_CTRL output; PVARP input; INTERVAL input; BLUE_LED output boolean
